simulink model "Cadlabproject"  (Simulink 7.7)
settings: Solver=ode45  StartTime=0.0  StopTime=1  RelTol=1e-3
undefined symbols (not defined in the file or in its folder): emfg
libraries: powerlib_extras x1
settings Model: Creator=mestan  LastModifiedBy=mestan

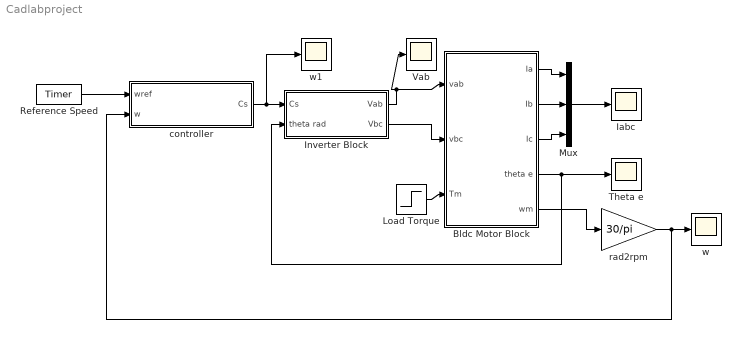
== system Cadlabproject ==
  Bldc Motor Block : Subsystem
  Iabc : Scope
      settings: YMin=-0.3  YMax=0.3  SaveName=ScopeData2
  Inverter Block : Subsystem
  Load Torque : Step  Time=0.2  After=0.2  SampleTime=0
  Mux : Mux  Inputs=3
  Reference Speed : powerlib_extras/Control  Blocks/Timer  SystemSampleTime=-1  t=[0 0.5]  e=[2000 1000]
  Theta e : Scope
      settings: YMin=1.00059  YMax=1.00067  SaveName=ScopeData3
  Vab : Scope
      settings: YMin=-20000  YMax=17500  SaveName=ScopeData4
  controller : Subsystem
  rad2rpm : Gain  Gain=30/pi
  w : Scope
      settings: TimeRange=1  YMin=950  YMax=2050
  w1 : Scope
      settings: TimeRange=0.4  YMin=725  YMax=1000
  wires:
  Load Torque/1 -> Bldc Motor Block/3(Tm)
  Inverter Block/2(Vbc) -> Bldc Motor Block/2(vbc)
  rad2rpm/1 -> w/1, controller/2(w)
  Bldc Motor Block/1(Ia) -> Mux/1
  Mux/1 -> Iabc/1
  Bldc Motor Block/2(Ib) -> Mux/2
  Bldc Motor Block/3(Ic) -> Mux/3
  Bldc Motor Block/4(theta e) -> Theta e/1, Inverter Block/2(theta rad)
  Bldc Motor Block/5(wm) -> rad2rpm/1
  controller/1(Cs) -> Inverter Block/1(Cs), w1/1
  Reference Speed/1 -> controller/1(wref)
  Inverter Block/1(Vab) -> Bldc Motor Block/1(vab), Vab/1

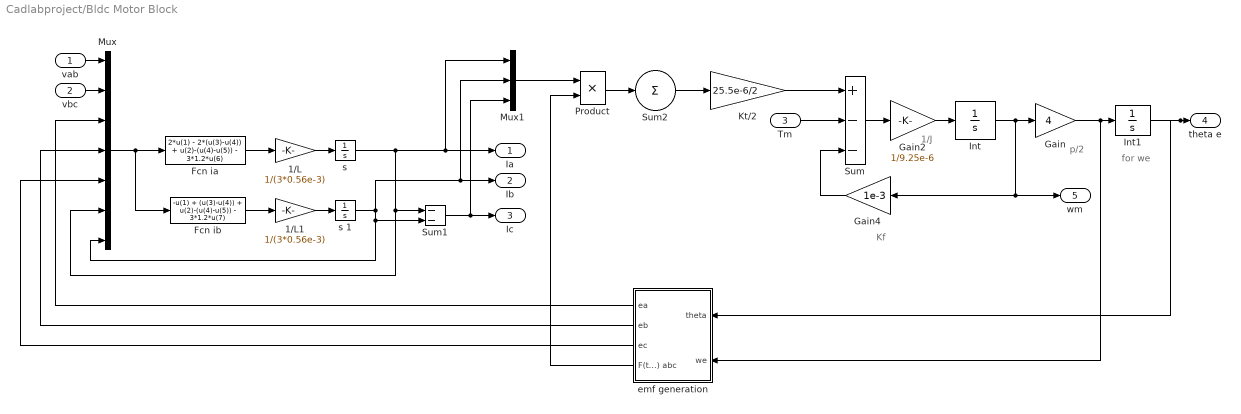
== system Cadlabproject/Bldc Motor Block ==
  note: 1/J
  note: Kf
  note: p/2
  note: for we
  vab : Inport
  vbc : Inport  Port=2
  Tm : Inport  Port=3
  1/L : Gain  Gain=1/(3*0.56e-3)  SaturateOnIntegerOverflow=on  OutDataTypeStr=Inherit: Same as input  ParamDataTypeStr=Inherit: Same as input
  1/L1 : Gain  Gain=1/(3*0.56e-3)  SaturateOnIntegerOverflow=on  OutDataTypeStr=Inherit: Same as input  ParamDataTypeStr=Inherit: Same as input
  Fcn ia : Fcn  Expr=2*u(1) - 2*(u(3)-u(4)) + u(2)-(u(4)-u(5)) - 3*1.2*u(6)
  Fcn ib : Fcn  Expr=-u(1) + (u(3)-u(4)) + u(2)-(u(4)-u(5)) - 3*1.2*u(7)
  Gain : Gain  Gain=4  SaturateOnIntegerOverflow=on  OutDataTypeStr=Inherit: Same as input  ParamDataTypeStr=Inherit: Same as input
  Gain2 : Gain  Gain=1/9.25e-6  SaturateOnIntegerOverflow=on  OutDataTypeStr=Inherit: Same as input  ParamDataTypeStr=Inherit: Same as input
  Gain4 : Gain  Gain=1e-3  SaturateOnIntegerOverflow=on  OutDataTypeStr=Inherit: Same as input  ParamDataTypeStr=Inherit: Same as input
  Int : Integrator
  Int1 : Integrator
  Kt/2 : Gain  Gain=25.5e-6/2  SaturateOnIntegerOverflow=on  OutDataTypeStr=Inherit: Same as input  ParamDataTypeStr=Inherit: Same as input
  Mux : Mux  Inputs=7
  Mux1 : Mux  Inputs=3
  Product : Product  SaturateOnIntegerOverflow=on  OutDataTypeStr=Inherit: Same as first input
  Sum : Sum  Inputs=+--  SaturateOnIntegerOverflow=on  InputSameDT=on  OutDataTypeStr=Inherit: Same as first input
  Sum1 : Sum  Inputs=--  SaturateOnIntegerOverflow=on
  Sum2 : Sum  Inputs=+  SaturateOnIntegerOverflow=on
  emf generation : Subsystem
  "s " : Integrator
  s 1 : Integrator
  Ia : Outport
  Ib : Outport  Port=2
  Ic : Outport  Port=3
  theta e : Outport  Port=4
  wm : Outport  Port=5
  wires:
  Fcn ia/1 -> 1/L/1
  Mux/1 -> Fcn ia/1, Fcn ib/1
  emf generation/1(ea) -> Mux/3
  emf generation/2(eb) -> Mux/4
  emf generation/3(ec) -> Mux/5
  vab/1 -> Mux/1
  vbc/1 -> Mux/2
  "s "/1 -> Mux/6, Sum1/1, Ia/1, Mux1/1
  1/L1/1 -> s 1/1
  Fcn ib/1 -> 1/L1/1
  s 1/1 -> Mux/7, Sum1/2, Mux1/2, Ib/1
  Sum1/1 -> Ic/1, Mux1/3
  1/L/1 -> "s "/1
  Sum2/1 -> Kt/2/1
  Product/1 -> Sum2/1
  Mux1/1 -> Product/1
  Int/1 -> Gain/1, Gain4/1, wm/1
  Gain2/1 -> Int/1
  Sum/1 -> Gain2/1
  Gain4/1 -> Sum/3
  Tm/1 -> Sum/2
  Kt/2/1 -> Sum/1
  emf generation/4(F(theta) abc) -> Product/2
  Gain/1 -> Int1/1, emf generation/2(we)
  Int1/1 -> theta e/1, emf generation/1(theta)

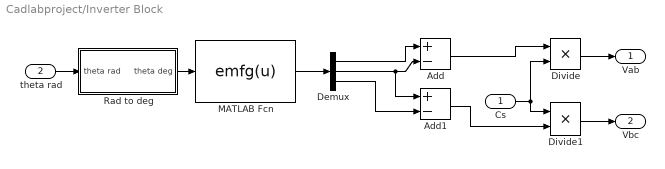
== system Cadlabproject/Inverter Block ==
  Cs : Inport
  theta rad : Inport  Port=2
  Add : Sum  Inputs=+-
  Add1 : Sum  Inputs=+-
  Demux : Demux  Outputs=3
  Divide : Product  Inputs=**
  Divide1 : Product  Inputs=**
  MATLAB Fcn : MATLABFcn  MATLABFcn=emfg(u)  OutputDimensions=3
  Rad to deg : Subsystem
  Vab : Outport
  Vbc : Outport  Port=2
  wires:
  theta rad/1 -> Rad to deg/1(theta rad)
  Rad to deg/1(theta deg) -> MATLAB Fcn/1
  MATLAB Fcn/1 -> Demux/1
  Demux/2 -> Add1/1, Add/2
  Demux/1 -> Add/1
  Demux/3 -> Add1/2
  Add/1 -> Divide/1
  Cs/1 -> Divide/2, Divide1/1
  Add1/1 -> Divide1/2
  Divide/1 -> Vab/1
  Divide1/1 -> Vbc/1

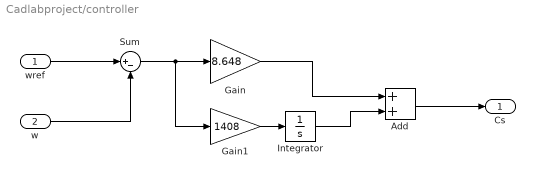
== system Cadlabproject/controller ==
  wref : Inport
  w : Inport  Port=2
  Add : Sum
  Gain : Gain  Gain=8.648
  Gain1 : Gain  Gain=1408
  Integrator : Integrator
  Sum : Sum  Inputs=|+-
  Cs : Outport
  wires:
  wref/1 -> Sum/1
  w/1 -> Sum/2
  Sum/1 -> Gain/1, Gain1/1
  Add/1 -> Cs/1
  Gain1/1 -> Integrator/1
  Gain/1 -> Add/1
  Integrator/1 -> Add/2

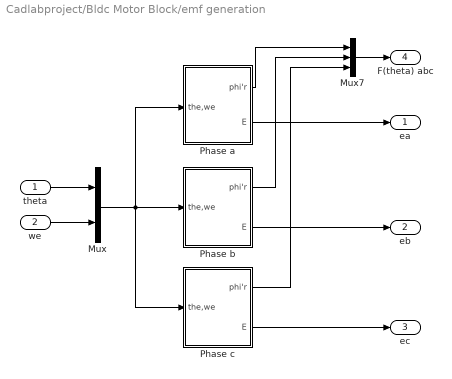
== system Cadlabproject/Bldc Motor Block/emf generation ==
  theta : Inport
  we : Inport  Port=2
  Mux : Mux  Inputs=2
  Mux7 : Mux  Inputs=3
  Phase a : Subsystem
  Phase b : Subsystem
  Phase c : Subsystem
  ea : Outport
  eb : Outport  Port=2
  ec : Outport  Port=3
  F(theta) abc : Outport  Port=4
  wires:
  Mux7/1 -> F(theta) abc/1
  Phase c/1(phi'r) -> Mux7/3
  Phase b/1(phi'r) -> Mux7/2
  Phase a/1(phi'r) -> Mux7/1
  Mux/1 -> Phase a/1(the,we), Phase b/1(the,we), Phase c/1(the,we)
  Phase a/2(E) -> ea/1
  Phase b/2(E) -> eb/1
  Phase c/2(E) -> ec/1
  theta/1 -> Mux/1
  we/1 -> Mux/2

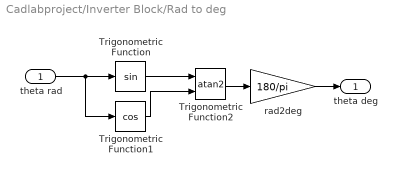
== system Cadlabproject/Inverter Block/Rad to deg ==
  theta rad : Inport
  Trigonometric Function : Trigonometry
  Trigonometric Function1 : Trigonometry  Operator=cos
  Trigonometric Function2 : Trigonometry  Operator=atan2
  rad2deg : Gain  Gain=180/pi  SaturateOnIntegerOverflow=on  OutDataTypeStr=Inherit: Same as input  ParamDataTypeStr=Inherit: Same as input
  theta deg : Outport
  wires:
  theta rad/1 -> Trigonometric Function/1, Trigonometric Function1/1
  Trigonometric Function/1 -> Trigonometric Function2/1
  Trigonometric Function1/1 -> Trigonometric Function2/2
  Trigonometric Function2/1 -> rad2deg/1
  rad2deg/1 -> theta deg/1

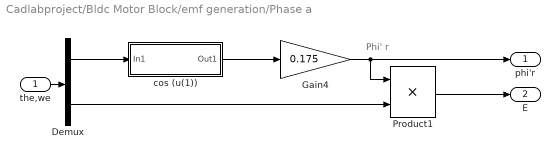
== system Cadlabproject/Bldc Motor Block/emf generation/Phase a ==
  note: Phi' r
  the,we : Inport
  Demux : Demux  Outputs=2
  Gain4 : Gain  Gain=0.175  SaturateOnIntegerOverflow=on  OutDataTypeStr=Inherit: Same as input  ParamDataTypeStr=Inherit: Same as input
  Product1 : Product  SaturateOnIntegerOverflow=on  OutDataTypeStr=Inherit: Same as first input
  cos (u(1)) : Subsystem
  phi'r : Outport
  E : Outport  Port=2
  wires:
  Gain4/1 -> Product1/1, phi'r/1
  Product1/1 -> E/1
  the,we/1 -> Demux/1
  Demux/2 -> Product1/2
  Demux/1 -> cos (u(1))/1(In1)
  cos (u(1))/1(Out1) -> Gain4/1

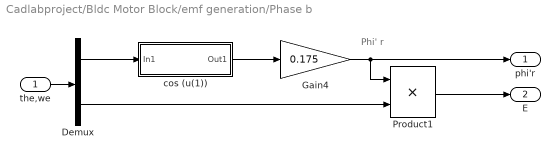
== system Cadlabproject/Bldc Motor Block/emf generation/Phase b ==
  note: Phi' r
  the,we : Inport
  Demux : Demux  Outputs=2
  Gain4 : Gain  Gain=0.175  SaturateOnIntegerOverflow=on  OutDataTypeStr=Inherit: Same as input  ParamDataTypeStr=Inherit: Same as input
  Product1 : Product  SaturateOnIntegerOverflow=on  OutDataTypeStr=Inherit: Same as first input
  cos (u(1)) : Subsystem
  phi'r : Outport
  E : Outport  Port=2
  wires:
  cos (u(1))/1(Out1) -> Gain4/1
  Demux/1 -> cos (u(1))/1(In1)
  Demux/2 -> Product1/2
  the,we/1 -> Demux/1
  Product1/1 -> E/1
  Gain4/1 -> phi'r/1, Product1/1

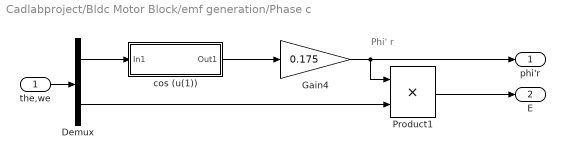
== system Cadlabproject/Bldc Motor Block/emf generation/Phase c ==
  note: Phi' r
  the,we : Inport
  Demux : Demux  Outputs=2
  Gain4 : Gain  Gain=0.175  SaturateOnIntegerOverflow=on  OutDataTypeStr=Inherit: Same as input  ParamDataTypeStr=Inherit: Same as input
  Product1 : Product  SaturateOnIntegerOverflow=on  OutDataTypeStr=Inherit: Same as first input
  cos (u(1)) : Subsystem
  phi'r : Outport
  E : Outport  Port=2
  wires:
  Gain4/1 -> Product1/1, phi'r/1
  Product1/1 -> E/1
  the,we/1 -> Demux/1
  Demux/2 -> Product1/2
  Demux/1 -> cos (u(1))/1(In1)
  cos (u(1))/1(Out1) -> Gain4/1

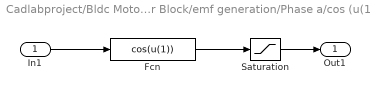
== system Cadlabproject/Bldc Motor Block/emf generation/Phase a/cos (u(1)) ==
  In1 : Inport
  Fcn : Fcn  Expr=cos(u(1))
  Saturation : Saturate  UpperLimit=0.8  LowerLimit=-0.8
  Out1 : Outport
  wires:
  In1/1 -> Fcn/1
  Fcn/1 -> Saturation/1
  Saturation/1 -> Out1/1

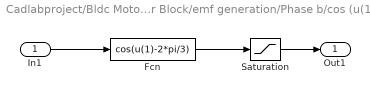
== system Cadlabproject/Bldc Motor Block/emf generation/Phase b/cos (u(1)) ==
  In1 : Inport
  Fcn : Fcn  Expr=cos(u(1)-2*pi/3)
  Saturation : Saturate  UpperLimit=0.8  LowerLimit=-0.8
  Out1 : Outport
  wires:
  In1/1 -> Fcn/1
  Fcn/1 -> Saturation/1
  Saturation/1 -> Out1/1

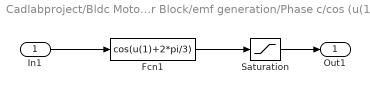
== system Cadlabproject/Bldc Motor Block/emf generation/Phase c/cos (u(1)) ==
  In1 : Inport
  Fcn1 : Fcn  Expr=cos(u(1)+2*pi/3)
  Saturation : Saturate  UpperLimit=0.8  LowerLimit=-0.8
  Out1 : Outport
  wires:
  In1/1 -> Fcn1/1
  Fcn1/1 -> Saturation/1
  Saturation/1 -> Out1/1
